simulink model "dynamic"  (R2023b)
settings: Solver=FixedStepAuto  StartTime=0.0  StopTime=10.0  FixedStep=1e-3  RelTol=1e-3
values from neighbouring files (symbols this model uses):
  a = mu / (2 * mu/r_mag - v_mag^2)    [q2032.m]    (also in q2120_sm.m = 10000)
  e = norm(e_vec)    [q2032.m]    (also in q2120_sm.m = 0.3)
  i_deg = rad2deg(i)    [q2032.m]    (also in q2120_sm.m = 45)
  Omega_deg = mod(rad2deg(Omega), 360)    [q2032.m]    (also in q2120_sm.m = 60)
  omega_deg = mod(rad2deg(omega), 360)    [q2032.m]    (also in q2120_sm.m = 30)
settings Model: Creator=asus  LastModifiedBy=asus

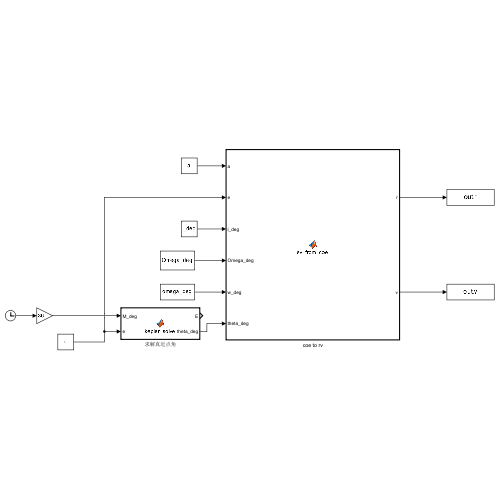
[thumbnail: Simulink's stored preview of the top-level diagram]
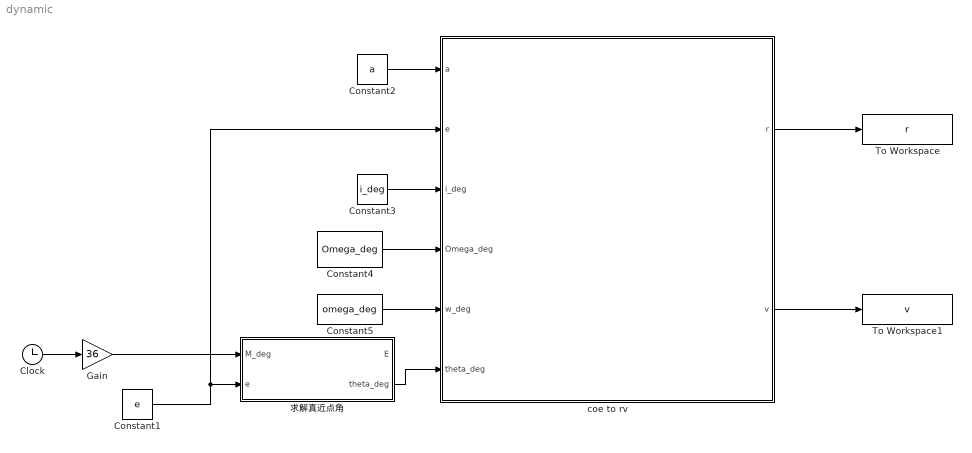
== system dynamic ==
  Clock : Clock
  Constant1 : Constant  Value=e
  Constant2 : Constant  Value=a
  Constant3 : Constant  Value=i_deg
  Constant4 : Constant  Value=Omega_deg
  Constant5 : Constant  Value=omega_deg
  Gain : Gain  Gain=36
  To Workspace : ToWorkspace  VariableName=r  SaveFormat=Timeseries  SampleTime=-1
  To Workspace1 : ToWorkspace  VariableName=v  SaveFormat=Timeseries  SampleTime=-1
  coe to rv : MATLAB Function  TreatAsAtomicUnit=on
  求解真近点角 : MATLAB Function  TreatAsAtomicUnit=on
  wires:
  求解真近点角/2(theta_deg) -> coe to rv/6(theta_deg)
  Constant1/1 -> 求解真近点角/2(e), coe to rv/2(e)
  Constant2/1 -> coe to rv/1(a)
  Gain/1 -> 求解真近点角/1(M_deg)
  Constant3/1 -> coe to rv/3(i_deg)
  Constant4/1 -> coe to rv/4(Omega_deg)
  Constant5/1 -> coe to rv/5(w_deg)
  coe to rv/1(r) -> To Workspace/1
  coe to rv/2(v) -> To Workspace1/1
  Clock/1 -> Gain/1

== matlab function dynamic/求解真近点角 ==
  data: E output; M_deg input; e input; theta_deg output
function [E, theta_deg] = kepler_solve(M_deg, e) 
    E = 0; 
    theta_deg = 0;
    M = mod(deg2rad(M_deg), 2*pi); 
    E = M;
    ratio = 1; 
    tol = 1e-8;
    while abs(ratio) > tol
        f = E - e*sin(E) - M;
        df = 1 - e*cos(E);
        ratio = f/df;
        E = E - ratio; 
    end
    theta = 2 * atan2(sqrt(1+e)*sin(E/2), sqrt(1-e)*cos(E/2));
    theta_deg = mod(rad2deg(theta), 360);
end

== matlab function dynamic/coe to rv ==
  data: a input; r output; e input; i_deg input; Omega_deg input; w_deg input; theta_deg input; v output
function [r, v] = sv_from_coe(a,e,i_deg,Omega_deg,w_deg,theta_deg)
% 输入 coe: [a (km), e, i (deg), Omega (deg), omega (deg), theta (deg)]
% 输出 r: 位置矢量 (km), v: 速度矢量 (km/s)

mu = 398600.4418; % 地球引力常数 km^3/s^2

i = deg2rad(i_deg);
Omega = deg2rad(Omega_deg); 
w = deg2rad(w_deg); 
theta = deg2rad(theta_deg);

p = a * (1 - e^2);
r_pqw = (p / (1 + e * cos(theta))) * [cos(theta); sin(theta); 0];
v_pqw = sqrt(mu/p) * [-sin(theta); e + cos(theta); 0];

R3_W = [cos(-Omega) sin(-Omega) 0; -sin(-Omega) cos(-Omega) 0; 0 0 1];
R1_i = [1 0 0; 0 cos(-i) sin(-i); 0 -sin(-i) cos(-i)];
R3_w = [cos(-w) sin(-w) 0; -sin(-w) cos(-w) 0; 0 0 1];

Q_p2i = (R3_w * R1_i * R3_W)'; 

r = Q_p2i * r_pqw;
v = Q_p2i * v_pqw;
end
